simulink model "Dadras"  (R2014b)
settings: Solver=ode45  StartTime=0.0  StopTime=10.0  RelTol=1e-3
values from neighbouring files (symbols this model uses):
  c = -1    [Run_Arneodo.m]    (also in Run_Chen.m = 25; Run_Chua_4D.m = -1.2; Run_Dadras.m = 2; Run_HindmarshRose.m = 1)
  e = 0.15    [Run_Aizawa.m]    (also in Run_Belousov_Zhabotinsky.m = 0.3; Run_Dadras.m = 9; Run_FitzHugh_Nagumo.m = 0.1)
  o = 2.7    [Run_Dadras.m]
  p = 3.0    (= 3)    [Run_Dadras.m]
  r = 1.7    [Run_Dadras.m]    (also in Run_HindmarshRose.m = 0.01; Run_Lorenz.m = 100; Script_Lorenz.m = 28)
undefined symbols (not defined in the file or in its folder): param
settings Model: Creator=Arek  LastModifiedBy=Arek

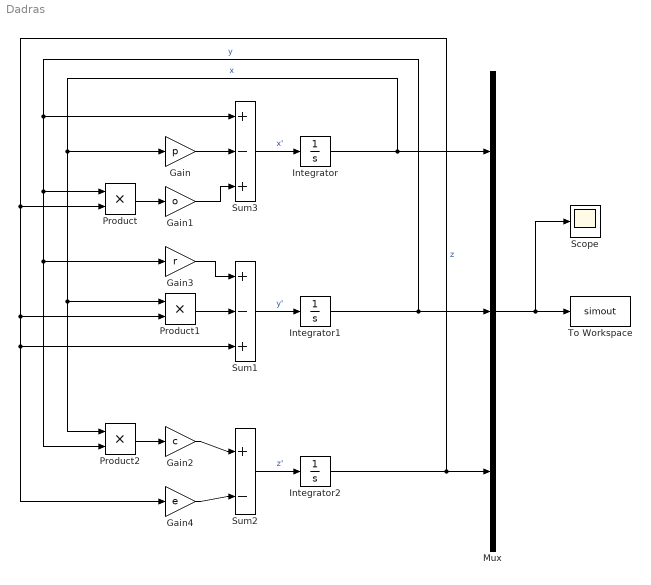
== system Dadras ==
  Gain : Gain  Gain=p
  Gain1 : Gain  Gain=o
  Gain2 : Gain  Gain=c
  Gain3 : Gain  Gain=r
  Gain4 : Gain  Gain=e
  Integrator : Integrator  InitialCondition=param.ic(1)
  Integrator1 : Integrator  InitialCondition=param.ic(2)
  Integrator2 : Integrator  InitialCondition=param.ic(3)
  Mux : Mux  Inputs=3
  Product : Product
  Product1 : Product
  Product2 : Product
  Scope : Scope
      settings: ShowLegends=on
  Sum1 : Sum  Inputs=+-+
  Sum2 : Sum  Inputs=+|-
  Sum3 : Sum  Inputs=+-+
  To Workspace : ToWorkspace  VariableName=simout  SaveFormat=Timeseries  SampleTime=-1
  wires:
  Integrator/1 -> Gain/1, Product2/1, Product1/1, Mux/1  "x"
  Sum1/1 -> Integrator1/1  "y'"
  Integrator1/1 -> Mux/2, Sum3/1, Product/1, Product2/2, Gain3/1  "y"
  Sum2/1 -> Integrator2/1  "z'"
  Integrator2/1 -> Product1/2, Gain4/1, Sum1/3, Product/2, Mux/3  "z"
  Mux/1 -> Scope/1, To Workspace/1
  Sum3/1 -> Integrator/1  "x'"
  Gain/1 -> Sum3/2
  Gain1/1 -> Sum3/3
  Product/1 -> Gain1/1
  Product1/1 -> Sum1/2
  Gain3/1 -> Sum1/1
  Gain2/1 -> Sum2/1
  Product2/1 -> Gain2/1
  Gain4/1 -> Sum2/2
